simulink model "PatientModelCL"  (R2019b)
settings: Solver=VariableStepAuto  StartTime=0.0  StopTime=30  FixedStep=0.1  MaxStep=1
model workspace (MAT data in the model file):
  C = tf
  C.IOSize_ = [1 1]
  C.Data_ = ltipack.tfdata
  C.Data_.num = {[-1 -2.2 -0.4]}
  C.Data_.den = {[0 1 2]}
  C.Data_.Delay.Input = 0
  C.Data_.Delay.Output = 0
  C.Data_.Delay.IO = 0
  C.Data_.Ts = 0
  params = Simulink.Parameter
  params.Value = [84.8056754884 23.1095578036 0.00886218404936 165.302304401 0 0.00346053352495 0 10.9713178124 98.2345782833 131.591642319 143.846149248 0 0 0 0 0 0 0 0 0]
  params.DataType = 'auto'
  params.Dimensions = [1 20]
libraries: cstblocks x1
settings Model: OrderedModelArguments=off  Creator=vjoukov  LastModifiedBy=zaria
settings SolverCC: InitialStep=.001
settings DataIOCC: ExternalInput=inputStruct  LoadExternalInput=on  ReturnWorkspaceOutputs=off
settings DebuggingCC: ArithmeticOperatorsInVariantConditions=warning
settings ModelReferenceCC: ModelReferenceMinAlgLoopOccurrences=on
settings SFSimCC: SimUseLocalCustomCode=off  CustomCodeUndefinedFunction=UseInterfaceOnly
settings RTWCC: RTWUseLocalCustomCode=off

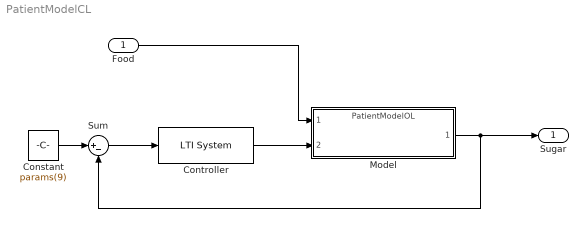
== system PatientModelCL ==
  Food : Inport
  Constant : Constant  Value=params(9)
  Controller : cstblocks/LTI System  sys=C  IC=[]
  Model : ModelReference  ModelNameDialog=PatientModelOL.slxp  ParameterArgumentNames=params  ParameterArgumentValues=params  UsingDefaultArgumentValue=0  ModelReferenceVersion=1.387  CopyOfModelProtected=on
  Sum : Sum  Inputs=|+-
  Sugar : Outport  VectorParamsAs1DForOutWhenUnconnected=off
  wires:
  Food/1 -> Model/1
  Model/1 -> Sum/2, Sugar/1
  Controller/1 -> Model/2
  Sum/1 -> Controller/1
  Constant/1 -> Sum/1
